simulink model "hexacopter_thomas"  (R2024b)
settings: Solver=ode3  StartTime=0.0  StopTime=inf  FixedStep=0.005  RelTol=1e-3
values from neighbouring files (symbols this model uses):
  A = [zeros(4),eye(4) ... (first row only)    [hexacopter_params.m]
  B = [0 0 0 0 ... (first row only)    [hexa.m]    (also in hexacopter_params.m = [zeros(4))
  body_params = [L,b,d,m,Ix,Iy,Iz,J_T]    [hexacopter_params.m]
  C = eye(8)    [hexacopter_params.m]
  g = 9.82    [hexacopter_params.m]
  K = place(A', C', desired_poles)'    [hexacopter_params.m]
  m = 2.5    [hexacopter_params.m]
  Simulation_params = [g,K_phi,K_theta,K_psi,K_x,K_y,K_z]    [hexacopter_params.m]
  T = [1, 1, 1, 1, 1, 1 ... (first row only)    [hexacopter_params.m]
  T_inv = pinv(T)    [hexacopter_params.m]
libraries: slpidlib x8, simulink_extras x3, aerolibutil x2, vrlib x2
(part 2 of 2)

== system hexacopter_thomas/Formatting/Euler to VR/Quaternion Normalization2 ==
  e0 : Inport
  1/2 : Gain  Gain=1/2  SaturateOnIntegerOverflow=on  OutDataTypeStr=Inherit: Same as input  ParamDataTypeStr=Inherit: Same as input
  Demux : Demux  Outputs=[1 3]
      settings: DisplayOption=none
  Mux : Mux  Inputs=2
  Product : Product  InputSameDT=on  SaturateOnIntegerOverflow=on  OutDataTypeStr=Inherit: Same as first input
  Trigonometric Function : Trigonometry
  Trigonometric Function1 : Trigonometry  Operator=cos
  e0_norm : Outport  VectorParamsAs1DForOutWhenUnconnected=off
  wires:
  Trigonometric Function1/1 -> Mux/1
  Demux/2 -> Product/2
  Demux/1 -> 1/2/1
  Mux/1 -> e0_norm/1
  Product/1 -> Mux/2
  Trigonometric Function/1 -> Product/1
  1/2/1 -> Trigonometric Function1/1, Trigonometric Function/1
  e0/1 -> Demux/1

== matlab function hexacopter_thomas/Subsystem/MATLAB Function1 ==
  data: eta input; state output; eta_dot input
function state = fcn(eta,eta_dot)

state = [eta(4);
         eta_dot(4);
         eta(5);
         eta_dot(5);
         eta(6);
         eta_dot(6);
         eta(3);
         eta_dot(3)];

== matlab function hexacopter_thomas/MATLAB Function ==
  data: thrusts input; motorspeeds output; params input
function motorspeeds = fcn(thrusts,params)

b = params(2); % Thrust coefficient [N/m^2]

% motorspeeds = sqrt(max(0,thrusts)/b);

nonneg_speeds = max(thrusts,0);
nonneg_indexes = find(thrusts<0);

for i=1:length(nonneg_indexes)
    idx = nonneg_indexes(i);
    if mod(idx,2)==0
        nonneg_speeds(idx-1) = nonneg_speeds(idx-1)+abs(thrusts(idx));
    else
        nonneg_speeds(idx+1) = nonneg_speeds(idx+1)+abs(thrusts(idx));
    end
end

motorspeeds = sqrt(nonneg_speeds/b);

motorspeeds = sqrt(max(0,thrusts)/b);

== matlab function hexacopter_thomas/Hexacopter model/Hexacopter dynamics ==
  data: nu_dot output; motorspeeds input; eta_dot input; eta input; hardware_params input; sim_params input
function nu_dot = fcn(motorspeeds,eta_dot,eta,hardware_params,sim_params)

L = hardware_params(1);
b = hardware_params(2);
d = hardware_params(3);
m = hardware_params(4);
Ix = hardware_params(5);
Iy = hardware_params(6);
Iz = hardware_params(7);
J_T = hardware_params(8);

F1 = b*motorspeeds(1)^2;
F2 = b*motorspeeds(2)^2;
F3 = b*motorspeeds(3)^2;
F4 = b*motorspeeds(4)^2;
F5 = b*motorspeeds(5)^2;
F6 = b*motorspeeds(6)^2;

tau1 = d*motorspeeds(1)^2;
tau2 = d*motorspeeds(2)^2;
tau3 = d*motorspeeds(3)^2;
tau4 = d*motorspeeds(4)^2;
tau5 = d*motorspeeds(5)^2;
tau6 = d*motorspeeds(6)^2;

U1 = F1+F2+F3+F4+F5+F6;
U2 = (F2-F1+(F3+F6-F4-F5)/2)*L;
U3 = (F3+F5-F4-F6)*L*sqrt(3)/2;
U4 = tau2+tau5+tau6-tau1-tau3-tau4;

g = sim_params(1);
K_phi = sim_params(2);
K_theta = sim_params(3);
K_psi = sim_params(4);
K_x = sim_params(5);
K_y = sim_params(6);
K_z = sim_params(7);

phi = eta(4);
theta = eta(5);
psi = eta(6);

x_dot = eta_dot(1);
y_dot = eta_dot(2); 
z_dot = eta_dot(3);
phi_dot = eta_dot(4);
theta_dot = eta_dot(5);
psi_dot = eta_dot(6);


Omega = motorspeeds(3)+motorspeeds(4)-motorspeeds(1)-motorspeeds(2);
max_omega = 1;  % Maximum yaw rate (in rad/s)
Omega = max(min(Omega, max_omega), -max_omega);  % Saturate Omega

nu_dot = zeros(6,1);
nu_dot(1) = (-U1*(cos(phi)*sin(theta)*cos(psi)+sin(phi)*sin(psi))-K_x*x_dot)/m;
nu_dot(2) = (-U1*(cos(phi)*sin(theta)*sin(psi)-sin(phi)*sin(psi))-K_y*y_dot)/m;
nu_dot(3) = -g+(U1*(cos(phi)*cos(theta))-K_z*z_dot)/m;
nu_dot(4) = (U2+(Iy-Iz)*theta_dot*psi_dot-J_T*theta_dot*Omega-K_phi*phi_dot)/Ix;
nu_dot(5) = (U3+(Iz-Ix)*phi_dot*psi_dot-J_T*phi_dot*Omega-K_theta*theta_dot)/Iy;
nu_dot(6) = (U4+(Ix-Iy)*phi_dot*theta_dot-K_psi*psi_dot)/Iz;

== matlab function hexacopter_thomas/Subsystem/MATLAB Function2 ==
  data: motorspeeds input; u output; hardware_params input
function u = fcn(motorspeeds,hardware_params)

L = hardware_params(1);
b = hardware_params(2);
d = hardware_params(3);

F1 = b*motorspeeds(1)^2;
F2 = b*motorspeeds(2)^2;
F3 = b*motorspeeds(3)^2;
F4 = b*motorspeeds(4)^2;
F5 = b*motorspeeds(5)^2;
F6 = b*motorspeeds(6)^2;

tau1 = d*motorspeeds(1)^2;
tau2 = d*motorspeeds(2)^2;
tau3 = d*motorspeeds(3)^2;
tau4 = d*motorspeeds(4)^2;
tau5 = d*motorspeeds(5)^2;
tau6 = d*motorspeeds(6)^2;

U1 = F1+F2+F3+F4+F5+F6;
U2 = (F2-F1+(F3+F6-F4-F5)/2)*L;
U3 = (F3+F5-F4-F6)*L*sqrt(3)/2;
U4 = tau2+tau5+tau6-tau1-tau3-tau4;

u = [U2;U3;U4;U1];

== matlab function hexacopter_thomas/Subsystem/MATLAB Function ==
  data: x_hat input; params input; motorspeeds input; out output
function out = h(x_hat,params,motorspeeds)

Ix = params(5);
Iy = params(6);
Iz = params(7);
J_T = params(8);

g = 9.82;

phi_dot = x_hat(2);
theta_dot = x_hat(4);
psi_dot = x_hat(6);

Omega = motorspeeds(3)+motorspeeds(4)-motorspeeds(1)-motorspeeds(2);
max_omega = 1;  % Maximum yaw rate (in rad/s)
Omega = max(min(Omega, max_omega), -max_omega);  % Saturate Omega

out = [zeros(4,1);
       (theta_dot*psi_dot*(Iy-Iz)-J_T*theta_dot*Omega)/Ix;
       (phi_dot*psi_dot*(Iz-Ix)-J_T*phi_dot*Omega)/Iy;
       phi_dot*theta_dot*(Ix-Iy)/Iz;
       -g];

% out = zeros(8,1);

== matlab function hexacopter_thomas/Fault Tolerant Control/Residual Validator/Single Motor Residual Validator ==
  data: r input; residual_results output; Mi input; Hi input
function residual_results = validate_residuals(r, Mi, Hi)
    r = r(5:8);
    residual_results = zeros(size(r));
    residual_results(r < Mi) = -1;
    residual_results(r > Hi) = 1;
end

== matlab function hexacopter_thomas/Fault Tolerant Control/Fault Isolation/MATLAB Function ==
  data: r input; fault_motor_id output; controllable output
function [fault_motor_id, controllable] = fault_lookup(r)
% r: 4x1 vector with values in {-1,0,1} for residuals 5..8

% Define fault patterns as rows in a matrix (faults x 4 residuals)
fault_patterns = [
   %r5  %r6  %r7  %r8
    1    0    1   -1;   % f1
   -1    0   -1   -1;   % f2
   -1   -1    1   -1;   % f3
    1    1    1   -1;   % f4
    1   -1   -1   -1;   % f5
   -1    1   -1   -1;   % f6
];

controllability = [1; 1; 0; 1; 0; 1];  % 1 = Yes, 0 = No

% Initialize outputs
fault_motor_id = 0;         % No fault by default
controllable = false;

for i = 1:size(fault_patterns,1)
    if isequal(r(:)', fault_patterns(i,:))
        fault_motor_id = i;
        controllable = logical(controllability(i));
        break;
    end
end

if all(r == 0)
    fault_motor_id = 0;
    controllable = true;
elseif fault_motor_id == 0
    fault_motor_id = -1;
    controllable = false;
end

end

== matlab function hexacopter_thomas/Fault Tolerant Control/MATLAB Function1 ==
  data: fault_motor_id input; T_out output; controllable input; T_in input
function T_out = recalculate_T(fault_motor_id, controllable, T_in)

if controllable == 1 && fault_motor_id == 0
    T_out = T_in;
    return;
end

if controllable == 0 && fault_motor_id == -1
    T_out = zeros(size(T_in));
    return;
end

T_out = T_in;
T_out(:, fault_motor_id) = 0;
% 
% disp("T_in")
% disp(T_in)
% disp("T_out")
% disp(T_out)
% disp("====")
